simulink model "CONTROLLER_LONG"  (R2015a)
settings: Solver=ode45  StartTime=0.0  StopTime=196  RelTol=1e-3
values from neighbouring files (symbols this model uses):
  A = [-0.0089 -0.1474 0 -9.75; -0.0216 -0.3601 5.9470 -0.151; 0 -0.00015 -0.0224 0.0006; 0 0 1 0]    [controller_design.m]
  B = [-2.682 9.748; 29 3.77; -3.847 -0.034; 0 0]    [controller_design.m]
  C = diag([1 1 1 1])    [controller_design.m]
  D = zeros(4,2)    [controller_design.m]
  K = place(A,B,p)    [controller_design.m]
  tht_tr = 6.30*(pi/180)    (= 0.109955742876)    [controller_design.m]
  u_tr = 155    [controller_design.m]
  w_tr = 0    [controller_design.m]
  XE_0 = 0    [constants.m]    (also in controller_design.m)
  ZE_0 = -2000    [constants.m]    (also in controller_design.m)
undefined symbols (not defined in the file or in its folder): Earth, magnitude, WGS84
libraries: aerolibtransform2 x1, simulink x1
settings Model: Creator=vinay  LastModifiedBy=vinay

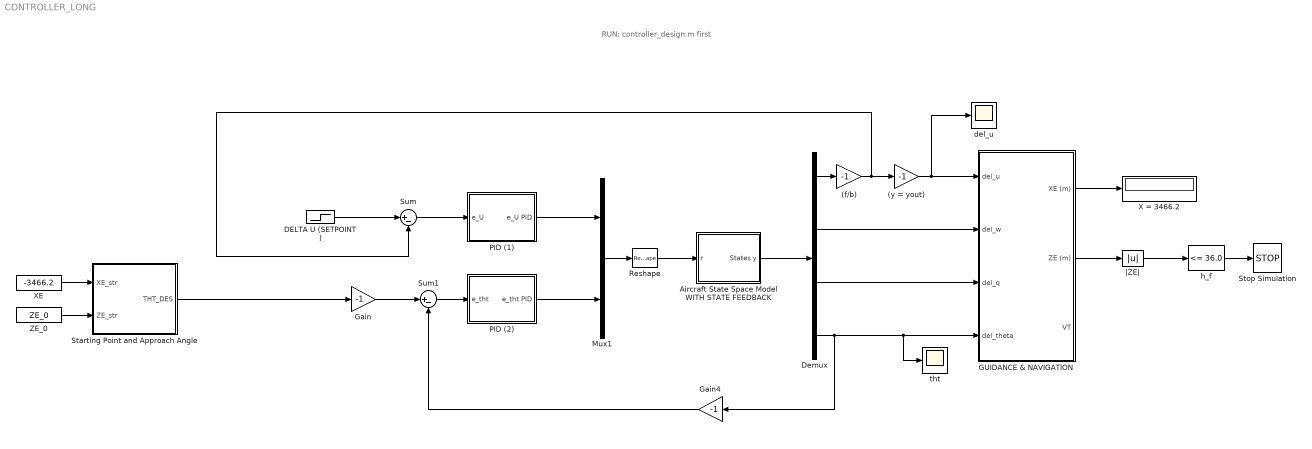
== system CONTROLLER_LONG ==
  note: RUN: controller_design.m first
  (f/b) : Gain  Gain=-1
  (y = yout) : Gain  Gain=-1
  Aircraft State Space Model WITH STATE FEEDBACK : Subsystem
  DELTA U (SETPOINT) : Step  After=24.3  SampleTime=0
  Demux : Demux
  "GUIDANCE & NAVIGATION " : Subsystem
  Gain : Gain  Gain=-1
  Gain4 : Gain  Gain=-1
  Mux1 : Mux  Inputs=2
  PID (1) : Subsystem
  PID (2) : Subsystem
  Reshape : Reshape  OutputDimensionality=Customize  OutputDimensions=[2,1]
  Starting Point and Approach Angle : Subsystem
  Stop Simulation : Stop
  Sum : Sum  Inputs=|+-
  Sum1 : Sum  Inputs=|+-
  X = 3466.2 : Display
  "XE " : Constant  Value=-3466.2
  ZE_0 : Constant  Value=ZE_0
  del_u : Scope
      settings: YMin=-1.225e+06  YMax=-800000
  h_f : simulink/Logic and Bit Operations/Compare To Constant  relop=<=  const=36.0  OutDataTypeStr=boolean
  tht : Scope
      settings: YMin=-57500  YMax=-10000
  |ZE| : Abs
  wires:
  Mux1/1 -> Reshape/1
  Reshape/1 -> Aircraft State Space Model WITH STATE FEEDBACK/1(r)
  Aircraft State Space Model WITH STATE FEEDBACK/1(States y) -> Demux/1
  ? -> ?
  Demux/1 -> (f/b)/1
  Gain/1 -> Sum1/1
  DELTA U (SETPOINT)/1 -> Sum/1
  Demux/4 -> "GUIDANCE & NAVIGATION "/4(del_theta), tht/1, Gain4/1
  Gain4/1 -> Sum1/2
  Sum/1 -> PID (1)/1(e_U)
  PID (1)/1(e_U PID) -> Mux1/1
  Sum1/1 -> PID (2)/1(e_tht)
  PID (2)/1(e_tht PID) -> Mux1/2
  Demux/2 -> "GUIDANCE & NAVIGATION "/2(del_w)
  Demux/3 -> "GUIDANCE & NAVIGATION "/3(del_q)
  "GUIDANCE & NAVIGATION "/2(ZE (m)) -> |ZE|/1
  |ZE|/1 -> h_f/1
  "XE "/1 -> Starting Point and Approach Angle/1(XE_str)
  ZE_0/1 -> Starting Point and Approach Angle/2(ZE_str)
  Starting Point and Approach Angle/1(THT_DES) -> Gain/1
  h_f/1 -> Stop Simulation/1
  (f/b)/1 -> Sum/2, (y = yout)/1
  (y = yout)/1 -> del_u/1, "GUIDANCE & NAVIGATION "/1(del_u)
  "GUIDANCE & NAVIGATION "/1(XE (m)) -> X = 3466.2/1

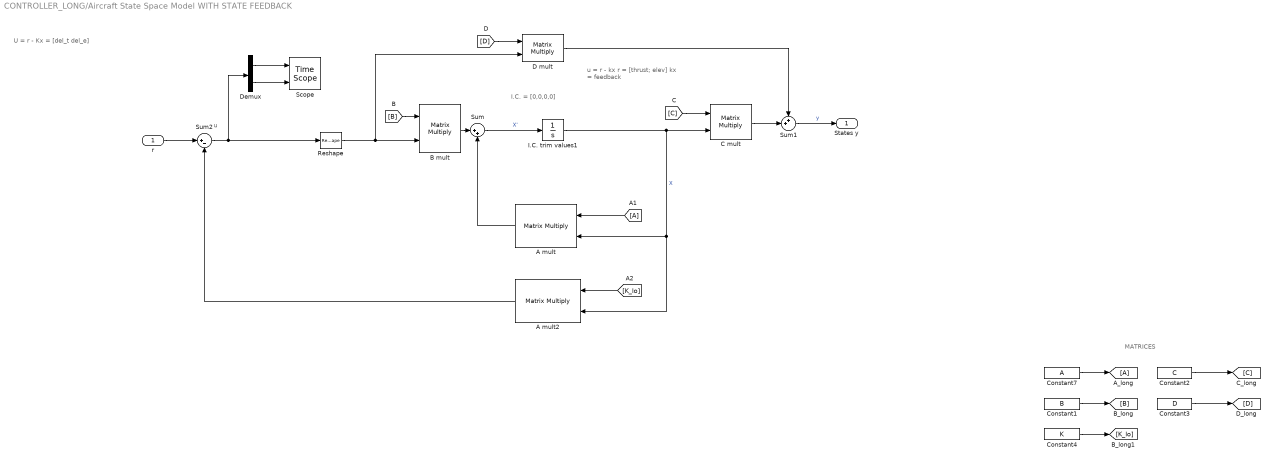
== system CONTROLLER_LONG/Aircraft State Space Model WITH STATE FEEDBACK ==
  note: u
  note: U = r - Kx = [del_t del_e]
  note: u = r - kx
      | r = [thrust; elev]
      | kx = feedback
  note: MATRICES
  note: I.C. = [0,0,0,0]
  r : Inport
  A mult : Product  Multiplication=Matrix(*)  RndMeth=Zero
  A mult2 : Product  Multiplication=Matrix(*)  RndMeth=Zero
  B mult : Product  Multiplication=Matrix(*)  RndMeth=Zero
  C mult : Product  Multiplication=Matrix(*)  RndMeth=Zero
  Constant1 : Constant  Value=B
  Constant2 : Constant  Value=C
  Constant3 : Constant  Value=D
  Constant4 : Constant  Value=K
  Constant7 : Constant  Value=A
  D mult : Product  Multiplication=Matrix(*)  RndMeth=Zero
  Demux : Demux  Outputs=2
  I.C. trim values1 : Integrator  InitialCondition=[0;0;0;0]
  Reshape : Reshape  OutputDimensionality=Customize  OutputDimensions=[2,1]
  Scope : TimeScope  NumInputPorts=2
  Sum : Sum  Inputs=|++
  Sum1 : Sum  Inputs=++|
  Sum2 : Sum  Inputs=|+-
  States y : Outport
  wires:
  Sum/1 -> I.C. trim values1/1  "X'"
  D mult/1 -> Sum1/1
  A mult/1 -> Sum/2
  [B] -> B mult/1
  [A] -> A mult/1
  [D] -> D mult/1
  [C] -> C mult/1
  Sum1/1 -> States y/1  "y"
  B mult/1 -> Sum/1
  C mult/1 -> Sum1/2
  Constant7/1 -> [A]
  Constant1/1 -> [B]
  Constant2/1 -> [C]
  Constant3/1 -> [D]
  Constant4/1 -> [K_lo]
  [K_lo] -> A mult2/1
  A mult2/1 -> Sum2/2
  r/1 -> Sum2/1
  Reshape/1 -> D mult/2, B mult/2
  I.C. trim values1/1 -> C mult/2, A mult2/2, A mult/2  "X"
  Sum2/1 -> Demux/1, Reshape/1
  Demux/1 -> Scope/1
  Demux/2 -> Scope/2

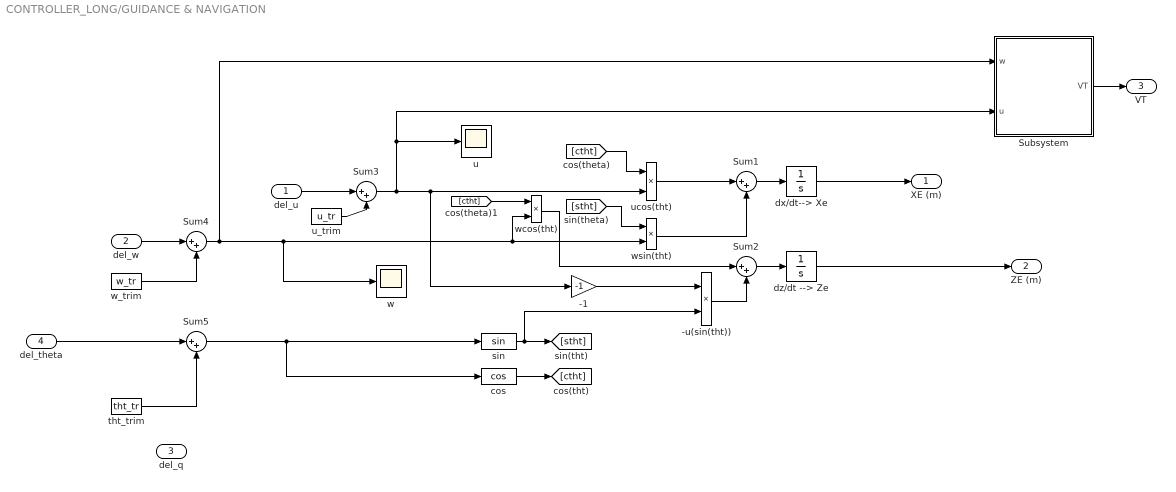
== system CONTROLLER_LONG/GUIDANCE & NAVIGATION  ==
  del_u : Inport
  del_w : Inport  Port=2
  del_q : Inport  Port=3
  del_theta : Inport  Port=4
  -1 : Gain  Gain=-1
  -u(sin(tht)) : Product
  Subsystem : Subsystem
  Sum{1..5} (5 alike) : Sum  Inputs=|++
  cos : Trigonometry  Operator=cos
  dx/dt--> Xe : Integrator  InitialCondition=XE_0
  dz/dt --> Ze : Integrator  InitialCondition=ZE_0
  sin : Trigonometry
  tht_trim : Constant  Value=tht_tr
  u : Scope
      settings: SaveName=ScopeData4
  u_trim : Constant  Value=u_tr
  ucos(tht) : Product
  w : Scope
      settings: SaveName=ScopeData5
  w_trim : Constant  Value=w_tr
  wcos(tht) : Product
  wsin(tht) : Product
  XE (m) : Outport
  ZE (m) : Outport  Port=2
  VT : Outport  Port=3
  wires:
  [stht] -> wsin(tht)/1
  wsin(tht)/1 -> Sum1/2
  dx/dt--> Xe/1 -> XE (m)/1
  ucos(tht)/1 -> Sum1/1
  dz/dt --> Ze/1 -> ZE (m)/1
  Sum1/1 -> dx/dt--> Xe/1
  Sum2/1 -> dz/dt --> Ze/1
  cos/1 -> [ctht]
  sin/1 -> -u(sin(tht))/2, [stht]
  wcos(tht)/1 -> Sum2/1
  [ctht] -> wcos(tht)/1
  -1/1 -> -u(sin(tht))/1
  [ctht] -> ucos(tht)/1
  -u(sin(tht))/1 -> Sum2/2
  tht_trim/1 -> Sum5/2
  del_u/1 -> Sum3/1
  Sum3/1 -> u/1, Subsystem/2(u), -1/1, ucos(tht)/2
  u_trim/1 -> Sum3/2
  del_w/1 -> Sum4/1
  Sum4/1 -> w/1, wcos(tht)/2, wsin(tht)/2, Subsystem/1(w)
  w_trim/1 -> Sum4/2
  del_theta/1 -> Sum5/1
  Sum5/1 -> cos/1, sin/1
  Subsystem/1(VT) -> VT/1

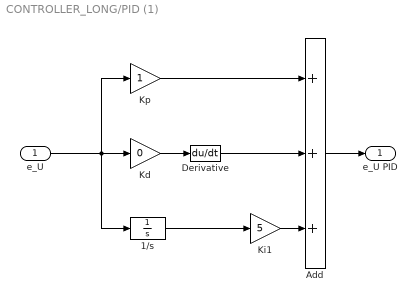
== system CONTROLLER_LONG/PID (1) ==
  e_U : Inport
  1/s : Integrator
  Add : Sum  Inputs=+++
  Derivative : Derivative
  Kd : Gain  Gain=0
  Ki1 : Gain  Gain=5
  Kp : Gain
  e_U PID : Outport
  wires:
  Add/1 -> e_U PID/1
  Kp/1 -> Add/1
  Ki1/1 -> Add/3
  e_U/1 -> 1/s/1, Kd/1, Kp/1
  Kd/1 -> Derivative/1
  Derivative/1 -> Add/2
  1/s/1 -> Ki1/1

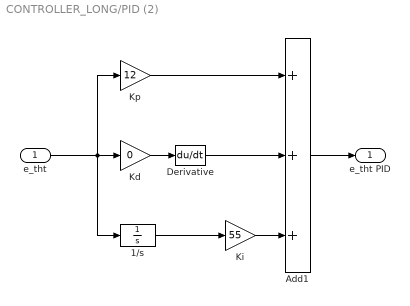
== system CONTROLLER_LONG/PID (2) ==
  e_tht : Inport
  1/s : Integrator
  Add1 : Sum  Inputs=+++
  Derivative : Derivative
  "Kd " : Gain  Gain=0
  "Ki " : Gain  Gain=55
  Kp : Gain  Gain=12
  e_tht PID : Outport
  wires:
  Add1/1 -> e_tht PID/1
  Kp/1 -> Add1/1
  e_tht/1 -> Kp/1, 1/s/1, "Kd "/1
  "Ki "/1 -> Add1/3
  "Kd "/1 -> Derivative/1
  Derivative/1 -> Add1/2
  1/s/1 -> "Ki "/1

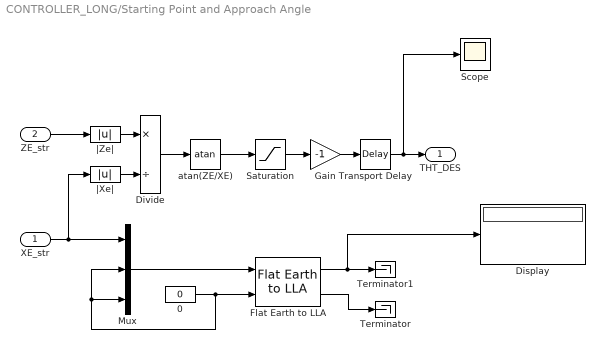
== system CONTROLLER_LONG/Starting Point and Approach Angle ==
  XE_str : Inport
  ZE_str : Inport  Port=2
  0 : Constant  Value=0
  Display : Display
  Divide : Product  Inputs=*/
  Flat Earth to LLA : aerolibtransform2/Flat Earth to LLA  units=Metric (MKS)  ptype=Earth (WGS84)  F=1/298.257223563  R=6378137  LL0=[45.457775 73.741389]  psi=h
  Gain : Gain  Gain=-1
  Mux : Mux  Inputs=3
  Saturation : Saturate  UpperLimit=0.5235  LowerLimit=-0.5235
  Scope : Scope
      settings: SaveName=ScopeData2
  Terminator : Terminator
  Terminator1 : Terminator
  Transport Delay : TransportDelay
  atan(ZE/XE) : Trigonometry  Operator=atan
  |Xe| : Abs
  |Ze| : Abs
  THT_DES : Outport
  wires:
  Mux/1 -> Flat Earth to LLA/1
  XE_str/1 -> |Xe|/1, Mux/1
  0/1 -> Mux/2, Mux/3, Flat Earth to LLA/2
  ZE_str/1 -> |Ze|/1
  |Ze|/1 -> Divide/1
  |Xe|/1 -> Divide/2
  Divide/1 -> atan(ZE/XE)/1
  Flat Earth to LLA/2 -> Terminator/1
  Saturation/1 -> Gain/1
  atan(ZE/XE)/1 -> Saturation/1
  Gain/1 -> Transport Delay/1
  Transport Delay/1 -> Scope/1, THT_DES/1
  Flat Earth to LLA/1 -> Display/1, Terminator1/1

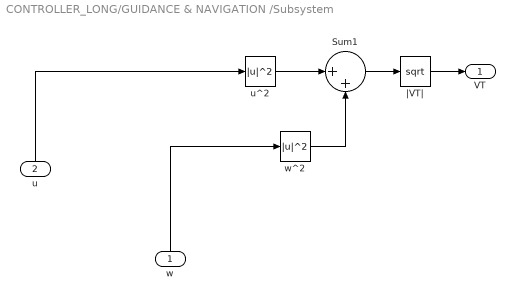
== system CONTROLLER_LONG/GUIDANCE & NAVIGATION /Subsystem ==
  w : Inport
  u : Inport  Port=2
  Sum1 : Sum  Inputs=|++
  u^2 : Math  Operator=magnitude^2  SaturateOnIntegerOverflow=on
  w^2 : Math  Operator=magnitude^2  SaturateOnIntegerOverflow=on
  |VT| : Sqrt  SaturateOnIntegerOverflow=on
  VT : Outport
  wires:
  Sum1/1 -> |VT|/1
  |VT|/1 -> VT/1
  u^2/1 -> Sum1/1
  w^2/1 -> Sum1/2
  w/1 -> w^2/1
  u/1 -> u^2/1
